simulink model "PhysicalModel"  (R2021a)
settings: Solver=VariableStepAuto  StartTime=0.0  StopTime=2  RelTol=1e-9
values from neighbouring files (symbols this model uses):
  Br = 2    [Fixed_Model.m]    (also in Matlab_Linear_Model.m; Matlab__Linear_Model.m = 20; Matlab__Linear_Model_2.m; Matlab__NonLinear_Model.m = 0.5)
  g = 9.81    [Fixed_Model.m]    (also in Matlab_Linear_Model.m; Matlab__Linear_Model.m; Matlab__Linear_Model_2.m; Matlab__NonLinear_Model.m)
  I = I1 + I2    (= 1.98633333333)    [Fixed_Model.m]    (also in Matlab_Linear_Model.m = 0.63768; Matlab__Linear_Model.m = 0.8924; Matlab__Linear_Model_2.m = 0.8924; Matlab__NonLinear_Model.m = 0.556904166667)
  l2x = (l1 + l2)/2 + l3x    (= 0.875)    [Fixed_Model.m]    (also in Matlab__Linear_Model.m = 0.65; Matlab__NonLinear_Model.m = 0.575)
  l3o = 0.3    [Fixed_Model.m]    (also in Matlab_Linear_Model.m = 0.15; Matlab__Linear_Model.m = 0.15; Matlab__Linear_Model_2.m = 0.15; Matlab__NonLinear_Model.m = 0.15)
  m2 = 2.5    [Fixed_Model.m]    (also in Matlab_Linear_Model.m = 1.4; Matlab__Linear_Model.m = 2; Matlab__Linear_Model_2.m = 2; Matlab__NonLinear_Model.m = 1.5)
  M2 = (F2*l2x)    (= -21.459375)    [Fixed_Model.m]    (also in Matlab__Linear_Model.m = -12.753; Matlab__NonLinear_Model.m = (F2*l2x*cos(theta)))
libraries: simulink x2
settings Model: Creator=DANI-TUF  LastModifiedBy=DANI-TUF

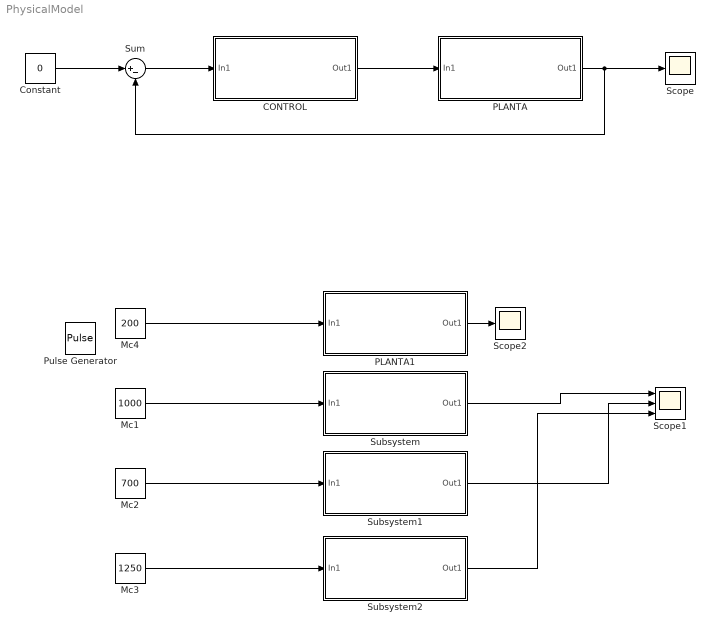
== system PhysicalModel ==
  CONTROL : Subsystem
  Constant : Constant  Value=0
  Mc1 : Constant  Value=1000
  Mc2 : Constant  Value=700
  Mc3 : Constant  Value=1250
  Mc4 : Constant  Value=200
  PLANTA : Subsystem
  PLANTA1 : Subsystem
  Pulse Generator : DiscretePulseGenerator  PulseType=Time based  Amplitude=10  Period=10  PulseWidth=10
  Scope : Scope
  Scope1 : Scope  NumInputPorts=3
  Scope2 : Scope
  Subsystem : Subsystem
  Subsystem1 : Subsystem
  Subsystem2 : Subsystem
  Sum : Sum  Inputs=|+-
  wires:
  Mc1/1 -> Subsystem/1(In1)
  Subsystem/1(Out1) -> Scope1/1
  Mc2/1 -> Subsystem1/1(In1)
  Subsystem1/1(Out1) -> Scope1/2
  Mc3/1 -> Subsystem2/1(In1)
  Subsystem2/1(Out1) -> Scope1/3
  CONTROL/1(Out1) -> PLANTA/1(In1)
  Sum/1 -> CONTROL/1(In1)
  Constant/1 -> Sum/1
  PLANTA/1(Out1) -> Sum/2, Scope/1
  PLANTA1/1(Out1) -> Scope2/1
  Mc4/1 -> PLANTA1/1(In1)

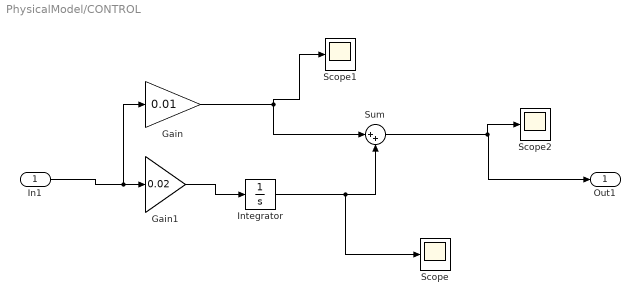
== system PhysicalModel/CONTROL ==
  In1 : Inport
  Gain : Gain  Gain=0.01
  Gain1 : Gain  Gain=0.02
  Integrator : Integrator
  Scope : Scope
  Scope1 : Scope
  Scope2 : Scope
  Sum : Sum  Inputs=|++
  Out1 : Outport
  wires:
  Sum/1 -> Scope2/1, Out1/1
  Gain1/1 -> Integrator/1
  Integrator/1 -> Scope/1, Sum/2
  In1/1 -> Gain/1, Gain1/1
  Gain/1 -> Sum/1, Scope1/1

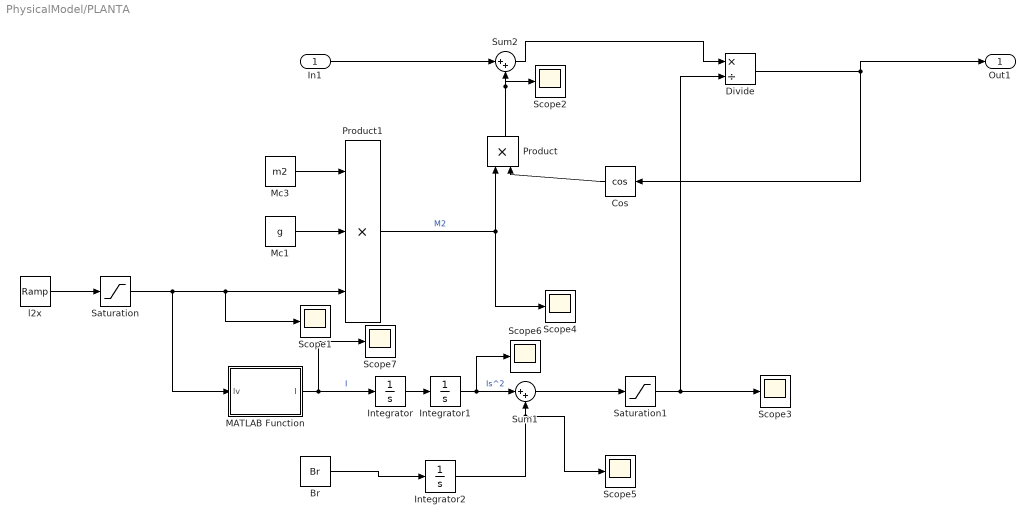
== system PhysicalModel/PLANTA ==
  In1 : Inport
  Br : Constant  Value=Br
  Cos : Trigonometry  Operator=cos
  Divide : Product  Inputs=*/
  Integrator : Integrator
  Integrator1 : Integrator  LimitOutput=on  UpperSaturationLimit=5.4
  Integrator2 : Integrator  LimitOutput=on  UpperSaturationLimit=2
  MATLAB Function : MATLAB Function  TreatAsAtomicUnit=on
  Mc1 : Constant  Value=g
  Mc3 : Constant  Value=m2
  Product : Product
  Product1 : Product  Inputs=3
  Saturation : Saturate  UpperLimit=l2x
  Saturation1 : Saturate  UpperLimit=inf  LowerLimit=1
  Scope{1..7} (7 alike) : Scope
  Sum1 : Sum  Inputs=|++
  Sum2 : Sum  Inputs=|++
  l2x : simulink/Sources/Ramp  slope=10  start=0  InitialOutput=l3o
  Out1 : Outport
  wires:
  Divide/1 -> Out1/1, Cos/1
  In1/1 -> Sum2/1
  Product/1 -> Scope2/1, Sum2/2
  Cos/1 -> Product/2
  Mc3/1 -> Product1/1
  Mc1/1 -> Product1/2
  l2x/1 -> Saturation/1
  Saturation/1 -> MATLAB Function/1(lv), Scope1/1, Product1/3
  Product1/1 -> Scope4/1, Product/1  "M2"
  Integrator/1 -> Integrator1/1
  MATLAB Function/1(I) -> Scope7/1, Integrator/1  "I"
  Integrator1/1 -> Scope6/1, Sum1/1  "Is^2"
  Br/1 -> Integrator2/1
  Sum1/1 -> Saturation1/1
  Sum2/1 -> Divide/1
  Saturation1/1 -> Scope3/1, Divide/2
  Integrator2/1 -> Scope5/1, Sum1/2

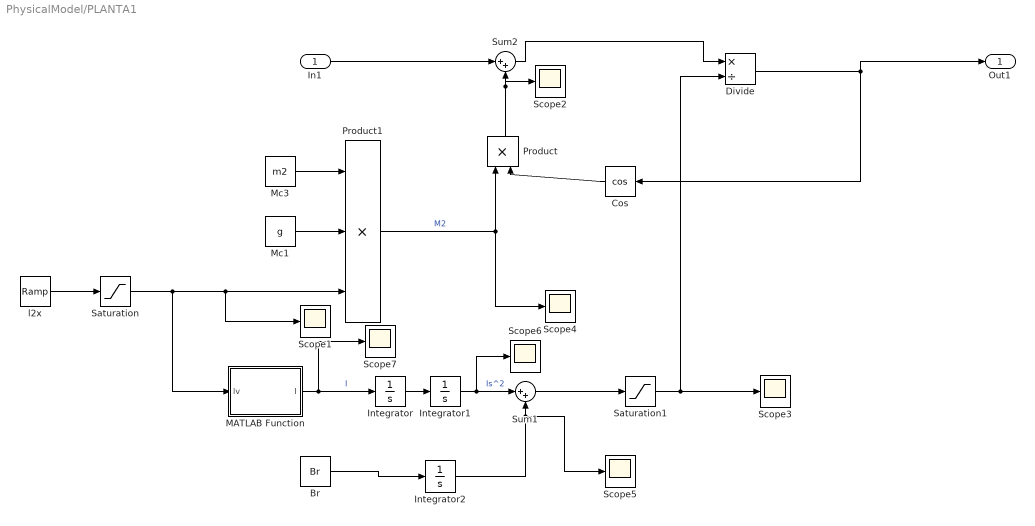
== system PhysicalModel/PLANTA1 ==
  In1 : Inport
  Br : Constant  Value=Br
  Cos : Trigonometry  Operator=cos
  Divide : Product  Inputs=*/
  Integrator : Integrator
  Integrator1 : Integrator  LimitOutput=on  UpperSaturationLimit=5.4
  Integrator2 : Integrator  LimitOutput=on  UpperSaturationLimit=2
  MATLAB Function : MATLAB Function  TreatAsAtomicUnit=on
  Mc1 : Constant  Value=g
  Mc3 : Constant  Value=m2
  Product : Product
  Product1 : Product  Inputs=3
  Saturation : Saturate  UpperLimit=l2x
  Saturation1 : Saturate  UpperLimit=inf  LowerLimit=1
  Scope{1..7} (7 alike) : Scope
  Sum1 : Sum  Inputs=|++
  Sum2 : Sum  Inputs=|++
  l2x : simulink/Sources/Ramp  slope=10  start=0  InitialOutput=l3o
  Out1 : Outport
  wires:
  Integrator2/1 -> Sum1/2, Scope5/1
  Saturation1/1 -> Divide/2, Scope3/1
  Sum2/1 -> Divide/1
  Sum1/1 -> Saturation1/1
  Br/1 -> Integrator2/1
  Integrator1/1 -> Sum1/1, Scope6/1  "Is^2"
  MATLAB Function/1(I) -> Integrator/1, Scope7/1  "I"
  Integrator/1 -> Integrator1/1
  Product1/1 -> Product/1, Scope4/1  "M2"
  Saturation/1 -> Product1/3, Scope1/1, MATLAB Function/1(lv)
  l2x/1 -> Saturation/1
  Mc1/1 -> Product1/2
  Mc3/1 -> Product1/1
  Cos/1 -> Product/2
  Product/1 -> Sum2/2, Scope2/1
  In1/1 -> Sum2/1
  Divide/1 -> Cos/1, Out1/1

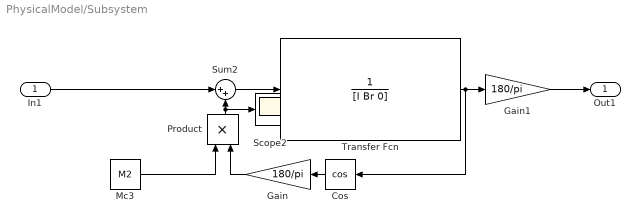
== system PhysicalModel/Subsystem ==
  In1 : Inport
  Cos : Trigonometry  Operator=cos
  Gain : Gain  Gain=180/pi
  Gain1 : Gain  Gain=180/pi
  Mc3 : Constant  Value=M2
  Product : Product
  Scope2 : Scope
  Sum2 : Sum  Inputs=|++
  Transfer Fcn : TransferFcn  Denominator=[I Br 0]
  Out1 : Outport
  wires:
  Cos/1 -> Gain/1
  Sum2/1 -> Transfer Fcn/1
  Gain/1 -> Product/2
  Mc3/1 -> Product/1
  Product/1 -> Scope2/1, Sum2/2
  In1/1 -> Sum2/1
  Gain1/1 -> Out1/1
  Transfer Fcn/1 -> Cos/1, Gain1/1

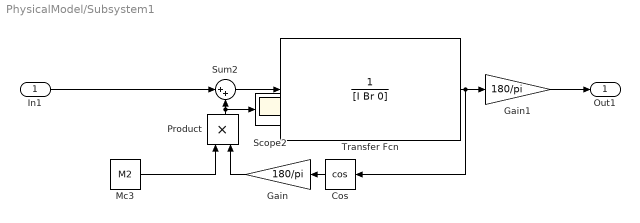
== system PhysicalModel/Subsystem1 ==
  In1 : Inport
  Cos : Trigonometry  Operator=cos
  Gain : Gain  Gain=180/pi
  Gain1 : Gain  Gain=180/pi
  Mc3 : Constant  Value=M2
  Product : Product
  Scope2 : Scope
  Sum2 : Sum  Inputs=|++
  Transfer Fcn : TransferFcn  Denominator=[I Br 0]
  Out1 : Outport
  wires:
  Transfer Fcn/1 -> Gain1/1, Cos/1
  Gain1/1 -> Out1/1
  In1/1 -> Sum2/1
  Product/1 -> Sum2/2, Scope2/1
  Mc3/1 -> Product/1
  Gain/1 -> Product/2
  Sum2/1 -> Transfer Fcn/1
  Cos/1 -> Gain/1

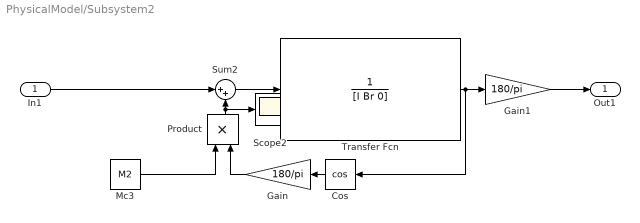
== system PhysicalModel/Subsystem2 ==
  In1 : Inport
  Cos : Trigonometry  Operator=cos
  Gain : Gain  Gain=180/pi
  Gain1 : Gain  Gain=180/pi
  Mc3 : Constant  Value=M2
  Product : Product
  Scope2 : Scope
  Sum2 : Sum  Inputs=|++
  Transfer Fcn : TransferFcn  Denominator=[I Br 0]
  Out1 : Outport
  wires:
  Cos/1 -> Gain/1
  Sum2/1 -> Transfer Fcn/1
  Gain/1 -> Product/2
  Mc3/1 -> Product/1
  Product/1 -> Scope2/1, Sum2/2
  In1/1 -> Sum2/1
  Gain1/1 -> Out1/1
  Transfer Fcn/1 -> Cos/1, Gain1/1

== matlab function PhysicalModel/PLANTA/MATLAB Function ==
  data: lv input; I output
function I = fcn(lv)
% Box dimensions
t1 = 0.2; % height of box 1 (m)
l1 = 0.35; % lenght of box 1 (m)

t2 = 0.12; % height of box 2 (m)
l2 = 0.2; % lenght of box 2 (m)

% IT SHOULD BE ON f(x)
l3o = 0.3; % Initial linear actuator lenght (m)
m1 = 4.5;   % Mass of box 1 (big box) (kg)
m2 = 2.5;   % Mass of box 2 (little box) (kg)

len = l1/2 + l2/2+lv+l3o;
I1 = (m1 * (t1^2 + l1^2))/12; % Rotational inertia of box 1 [Kg*m^2]
I2 = (m2 * (t2^2 + l2^2))/12 + (m2 * len^2) ; % Rotational inertia of box 2 [Kg*m^2]

I = I1 + I2; % Rotational Inertia #CHECK

== matlab function PhysicalModel/PLANTA1/MATLAB Function ==
  data: lv input; I output
function I = fcn(lv)
% Box dimensions
t1 = 0.2; % height of box 1 (m)
l1 = 0.35; % lenght of box 1 (m)

t2 = 0.12; % height of box 2 (m)
l2 = 0.2; % lenght of box 2 (m)

% IT SHOULD BE ON f(x)
l3o = 0.3; % Initial linear actuator lenght (m)
m1 = 4.5;   % Mass of box 1 (big box) (kg)
m2 = 2.5;   % Mass of box 2 (little box) (kg)

len = l1/2 + l2/2+lv+l3o;
I1 = (m1 * (t1^2 + l1^2))/12; % Rotational inertia of box 1 [Kg*m^2]
I2 = (m2 * (t2^2 + l2^2))/12 + (m2 * len^2) ; % Rotational inertia of box 2 [Kg*m^2]

I = I1 + I2; % Rotational Inertia #CHECK
